simulink model "three_phase_resistive_thermal_model"  (R2015a)
settings: Solver=ode45  StartTime=0.0  StopTime=10.0  RelTol=1e-3
libraries: fl_lib x40
settings Model: Creator=Caner  LastModifiedBy=Caner

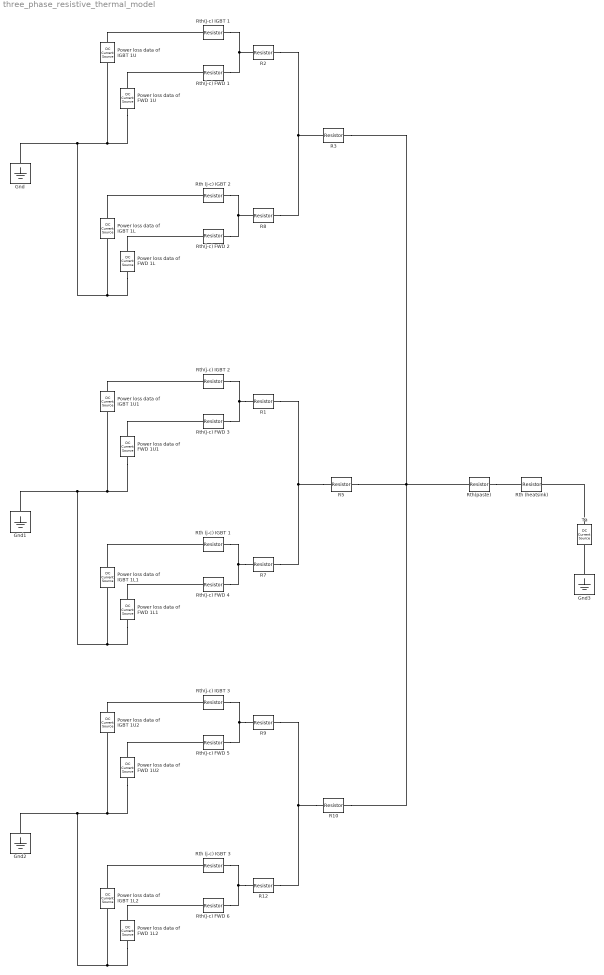
== system three_phase_resistive_thermal_model ==
  Gnd{,1..3} (4 alike) : fl_lib/Electrical/Electrical Elements/Electrical Reference
  Power loss data of FWD 1L : fl_lib/Electrical/Electrical Sources/DC Current Source  i0=1 A
  Power loss data of FWD 1L1 : fl_lib/Electrical/Electrical Sources/DC Current Source  i0=1 A
  Power loss data of FWD 1L2 : fl_lib/Electrical/Electrical Sources/DC Current Source  i0=1 A
  Power loss data of FWD 1U : fl_lib/Electrical/Electrical Sources/DC Current Source  i0=1 A
  Power loss data of FWD 1U1 : fl_lib/Electrical/Electrical Sources/DC Current Source  i0=1 A
  Power loss data of FWD 1U2 : fl_lib/Electrical/Electrical Sources/DC Current Source  i0=1 A
  Power loss data of IGBT 1L : fl_lib/Electrical/Electrical Sources/DC Current Source  i0=1 A
  Power loss data of IGBT 1L1 : fl_lib/Electrical/Electrical Sources/DC Current Source  i0=1 A
  Power loss data of IGBT 1L2 : fl_lib/Electrical/Electrical Sources/DC Current Source  i0=1 A
  Power loss data of IGBT 1U : fl_lib/Electrical/Electrical Sources/DC Current Source  i0=1 A
  Power loss data of IGBT 1U1 : fl_lib/Electrical/Electrical Sources/DC Current Source  i0=1 A
  Power loss data of IGBT 1U2 : fl_lib/Electrical/Electrical Sources/DC Current Source  i0=1 A
  R{1..3,5,7..10,12} (9 alike) : fl_lib/Electrical/Electrical Elements/Resistor  R=1 Ohm  i_specify=off  i_priority=High  i=0 A  v_specify=off  v_priority=High  v=0 V
  Rth (heatsink) : fl_lib/Electrical/Electrical Elements/Resistor  R=1 Ohm  i_specify=off  i_priority=High  i=0 A  v_specify=off  v_priority=High  v=0 V
  Rth (j-c) IGBT 1 : fl_lib/Electrical/Electrical Elements/Resistor  R=1 Ohm  i_specify=off  i_priority=High  i=0 A  v_specify=off  v_priority=High  v=0 V
  Rth (j-c) IGBT 2 : fl_lib/Electrical/Electrical Elements/Resistor  R=1 Ohm  i_specify=off  i_priority=High  i=0 A  v_specify=off  v_priority=High  v=0 V
  Rth (j-c) IGBT 3 : fl_lib/Electrical/Electrical Elements/Resistor  R=1 Ohm  i_specify=off  i_priority=High  i=0 A  v_specify=off  v_priority=High  v=0 V
  Rth(j-c) FWD {1..6} (6 alike) : fl_lib/Electrical/Electrical Elements/Resistor  R=1 Ohm  i_specify=off  i_priority=High  i=0 A  v_specify=off  v_priority=High  v=0 V
  Rth(j-c) IGBT 1 : fl_lib/Electrical/Electrical Elements/Resistor  R=1 Ohm  i_specify=off  i_priority=High  i=0 A  v_specify=off  v_priority=High  v=0 V
  Rth(j-c) IGBT 2 : fl_lib/Electrical/Electrical Elements/Resistor  R=1 Ohm  i_specify=off  i_priority=High  i=0 A  v_specify=off  v_priority=High  v=0 V
  Rth(j-c) IGBT 3 : fl_lib/Electrical/Electrical Elements/Resistor  R=1 Ohm  i_specify=off  i_priority=High  i=0 A  v_specify=off  v_priority=High  v=0 V
  Rth(paste) : fl_lib/Electrical/Electrical Elements/Resistor  R=1 Ohm  i_specify=off  i_priority=High  i=0 A  v_specify=off  v_priority=High  v=0 V
  "Ta " : fl_lib/Electrical/Electrical Sources/DC Current Source  i0=1 A
  connections:
  Power loss data of IGBT 1U/LConn1 -- Rth(j-c) IGBT 1/LConn1
  Rth(j-c) IGBT 1/RConn1 -- Rth(j-c) FWD 1/RConn1 -- R2/LConn1
  R2/RConn1 -- R8/RConn1 -- R3/LConn1
  Power loss data of IGBT 1L/RConn1 -- Power loss data of FWD 1U/RConn1 -- Power loss data of IGBT 1U/RConn1 -- Gnd/LConn1 -- Power loss data of FWD 1L/RConn1
  Power loss data of FWD 1U/LConn1 -- Rth(j-c) FWD 1/LConn1
  Power loss data of FWD 1L/LConn1 -- Rth(j-c) FWD 2/LConn1
  Power loss data of IGBT 1L/LConn1 -- Rth (j-c) IGBT 2/LConn1
  Rth (j-c) IGBT 2/RConn1 -- Rth(j-c) FWD 2/RConn1 -- R8/LConn1
  R1/LConn1 -- Rth(j-c) IGBT 2/RConn1 -- Rth(j-c) FWD 3/RConn1
  R5/LConn1 -- R1/RConn1 -- R7/RConn1
  Power loss data of IGBT 1L1/RConn1 -- Power loss data of FWD 1U1/RConn1 -- Power loss data of IGBT 1U1/RConn1 -- Gnd1/LConn1 -- Power loss data of FWD 1L1/RConn1
  R7/LConn1 -- Rth (j-c) IGBT 1/RConn1 -- Rth(j-c) FWD 4/RConn1
  Power loss data of FWD 1U1/LConn1 -- Rth(j-c) FWD 3/LConn1
  Power loss data of IGBT 1U1/LConn1 -- Rth(j-c) IGBT 2/LConn1
  R5/RConn1 -- R3/RConn1 -- R10/RConn1 -- Rth(paste)/LConn1
  Power loss data of IGBT 1L1/LConn1 -- Rth (j-c) IGBT 1/LConn1
  Power loss data of FWD 1L1/LConn1 -- Rth(j-c) FWD 4/LConn1
  R9/LConn1 -- Rth(j-c) IGBT 3/RConn1 -- Rth(j-c) FWD 5/RConn1
  R10/LConn1 -- R9/RConn1 -- R12/RConn1
  Power loss data of IGBT 1L2/RConn1 -- Power loss data of FWD 1U2/RConn1 -- Power loss data of IGBT 1U2/RConn1 -- Gnd2/LConn1 -- Power loss data of FWD 1L2/RConn1
  R12/LConn1 -- Rth (j-c) IGBT 3/RConn1 -- Rth(j-c) FWD 6/RConn1
  Power loss data of FWD 1U2/LConn1 -- Rth(j-c) FWD 5/LConn1
  Power loss data of IGBT 1U2/LConn1 -- Rth(j-c) IGBT 3/LConn1
  Power loss data of IGBT 1L2/LConn1 -- Rth (j-c) IGBT 3/LConn1
  Power loss data of FWD 1L2/LConn1 -- Rth(j-c) FWD 6/LConn1
  Rth(paste)/RConn1 -- Rth (heatsink)/LConn1
  "Ta "/RConn1 -- Rth (heatsink)/RConn1
  Gnd3/LConn1 -- "Ta "/LConn1
